simulink model "Part_b"  (R2021b)
settings: Solver=FixedStepDiscrete  StartTime=0.0  StopTime=inf  RelTol=1e-3
undefined symbols (not defined in the file): D4
libraries: androiduilib x8, androidsensorlib x2, androidaudiovideolib x1, androidcommunicationlib x1, fuzblock x1
settings Model: Creator=Nishikant Parmar  LastModifiedBy=Nishikant Parmar
settings OptimizationCC: EnhancedBackFolding=on  PassReuseOutputArgsAs=Individual arguments  ZeroExternalMemoryAtStartup=off  ZeroInternalMemoryAtStartup=off  MaxStackSize=64  OptimizeBlockOrder=speed  DifferentSizesBufferReuse=on  OptimizationCustomize=off  EfficientTunableParamExpr=on
settings DebuggingCC: ParameterTunabilityLossMsg=error
settings HardwareCC: ProdBitPerPointer=32  ProdBitPerSizeT=32  ProdBitPerPtrDiffT=32  ProdLargestAtomicInteger=Long  ProdLargestAtomicFloat=Double  ProdWordSize=32  ProdHWDeviceType=ARM Compatible->ARM Cortex  UseEmbeddedCoderFeatures=off  UseSimulinkCoderFeatures=off
settings SFSimCC: MATLABDynamicMemAlloc=off
settings RTWCC: Description=Embedded Coder  SystemTargetFile=ert.tlc  HardwareBoard=Android Device  TLCOptions="-aInlineSetEventsForThisBaseRateFcn=TLC_FALSE -aSuppressMultiTaskScheduler=TLC_FALSE  -aRateBasedStepFcn=0"  TemplateMakefile=ert_default_tmf  RTWVerbose=off  Toolchain=Android SDK/NDK Tools
settings CodeAppCC: ForceParamTrailComments=on  IgnoreCustomStorageClasses=off  OperatorAnnotations=on  SimulinkDataObjDesc=on  SFDataObjDesc=on  InsertBlockDesc=on
settings ERTTargetCC: SupportNonInlinedSFcns=on

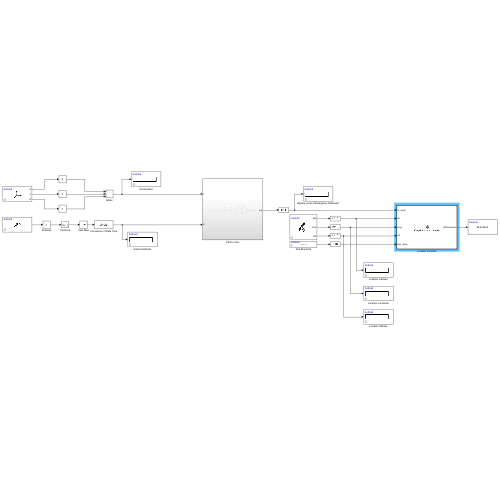
[thumbnail: Simulink's stored preview of the top-level diagram]
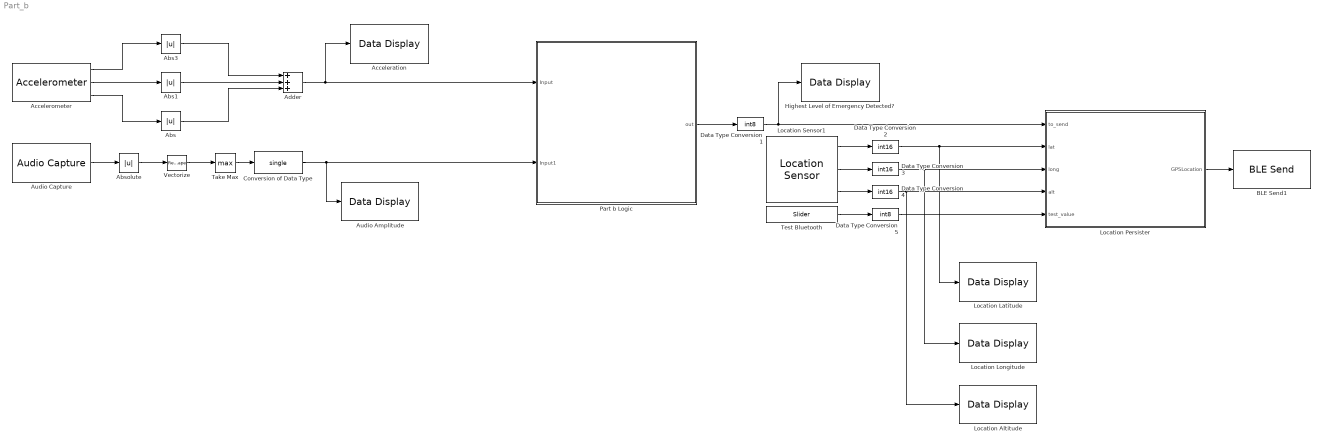
== system Part_b ==
  Abs : Abs
  Abs1 : Abs
  Abs3 : Abs
  Absolute : Abs
  Acceleration : androiduilib/Data Display  DataDisplayId=Part_b/Acceleration  Format=Float  Precision=6  SimulateUsing=Code generation  blockPlatform=Android
      settings: SourceProductBaseCode=ANDROID
  Accelerometer : androidsensorlib/Accelerometer  OutputVector=off  SampleTime=0.1  BlockPlatform=Android
      settings: SourceProductBaseCode=ANDROID
  Adder : Sum  Inputs=+++
  Audio Amplitude : androiduilib/Data Display  DataDisplayId=Part_b/Audio_Amplitude  Format=Float  Precision=6  SimulateUsing=Code generation  blockPlatform=Android
      settings: SourceProductBaseCode=ANDROID
  Audio Capture : androidaudiovideolib/Audio Capture  SampleFreq=44100  FrameSize=4410  SampleTime=0.1  SimulateUsing=Code generation  DeviceStr=0  QueueDuration=0  BlockPlatform=Android  AudioSamplingFreq=44100
      settings: SourceProductBaseCode=ANDROID
  BLE Send1 : androidcommunicationlib/BLE Send  DeviceMode=Peripheral (Server)  BluetoothAddress=D4:8A:39:6B:66:89  CharUUID=00002a05-0000-1000-8000-00805f9b34fb  ServiceUUID=00001801-0000-1000-8000-00805f9b34fb  device=Nishikant's Galaxy M31s  character=Generic Attribute\Service Changed  CustomService=off  ServiceName=Heart Rate  CharacteristicName="Heart Rate  Measurement"  CustomServiceUUID=<Enter Service UUID>  CustomCharUUID=<Enter Characteristic UUID>  charseruuid=00001801-0000-1000-8000-00805f9b34fb\00002a05-0000-1000-8000-00805f9b34fb  seruuid=00001810-0000-1000-8000-00805f9b34fb  chruuid=00002a37-0000-1000-8000-00805f9b34fb  PeripheralService=0000180d-0000-1000-8000-00805f9b34fb  PeripheralCharacteristic=00002a37-0000-1000-8000-00805f9b34fb  BLEId=Part_b/BLE_Send1  Devicename=Nishikant's Galaxy M31s  IsCustomService=0  Size=-1
      settings: SourceProductBaseCode=ANDROID
  Conversion of Data Type : DataTypeConversion  OutDataTypeStr=single
  Data Type Conversion1 : DataTypeConversion  OutDataTypeStr=int8
  Data Type Conversion2 : DataTypeConversion  OutDataTypeStr=int16
  Data Type Conversion3 : DataTypeConversion  OutDataTypeStr=int16
  Data Type Conversion4 : DataTypeConversion  OutDataTypeStr=int16
  Data Type Conversion5 : DataTypeConversion  OutDataTypeStr=int8
  Highest Level of Emergency Detected? : androiduilib/Data Display  DataDisplayId=Part_b/Highest_Level_of_Emergency_Detected?  Format=Float  Precision=6  SimulateUsing=Code generation  blockPlatform=Android
      settings: SourceProductBaseCode=ANDROID
  Location Altitude : androiduilib/Data Display  DataDisplayId=Part_b/Location_Altitude  Format=Float  Precision=6  SimulateUsing=Code generation  blockPlatform=Android
      settings: SourceProductBaseCode=ANDROID
  Location Latitude : androiduilib/Data Display  DataDisplayId=Part_b/Location_Latitude  Format=Float  Precision=6  SimulateUsing=Code generation  blockPlatform=Android
      settings: SourceProductBaseCode=ANDROID
  Location Longitude : androiduilib/Data Display  DataDisplayId=Part_b/Location_Longitude  Format=Float  Precision=6  SimulateUsing=Code generation  blockPlatform=Android
      settings: SourceProductBaseCode=ANDROID
  Location Persister : MATLAB Function  TreatAsAtomicUnit=on
  Location Sensor1 : androidsensorlib/Location Sensor  OutputVector=off  SampleTime=0.1  BlockPlatform=Android
      settings: SourceProductBaseCode=ANDROID
  Part b Logic : Subsystem
  Take Max : MinMax  Function=max
  Test Bluetooth : androiduilib/Slider  Min=-127  Value=0  Max=128  Resolution=1  SliderId=Part_b/Test_Bluetooth  SampleTime=0.1  BlockPlatform=Android
      settings: SourceProductBaseCode=ANDROID
  Vectorize : Reshape
  wires:
  Audio Capture/1 -> Absolute/1
  Accelerometer/1 -> Abs3/1
  Accelerometer/2 -> Abs1/1
  Accelerometer/3 -> Abs/1
  Abs3/1 -> Adder/1
  Abs1/1 -> Adder/2
  Abs/1 -> Adder/3
  Absolute/1 -> Vectorize/1
  Vectorize/1 -> Take Max/1
  Adder/1 -> Acceleration/1, Part b Logic/1(Input)
  Take Max/1 -> Conversion of Data Type/1
  Conversion of Data Type/1 -> Part b Logic/2(Input1), Audio Amplitude/1
  Data Type Conversion4/1 -> Location Altitude/1, Location Persister/4(alt)
  Location Sensor1/2 -> Data Type Conversion3/1
  Data Type Conversion3/1 -> Location Longitude/1, Location Persister/3(long)
  Test Bluetooth/1 -> Data Type Conversion5/1
  Location Persister/1(GPSLocation) -> BLE Send1/1
  Data Type Conversion1/1 -> Highest Level of Emergency Detected?/1, Location Persister/1(to_send)
  Data Type Conversion5/1 -> Location Persister/5(test_value)
  Data Type Conversion2/1 -> Location Latitude/1, Location Persister/2(lat)
  Part b Logic/1(out) -> Data Type Conversion1/1
  Location Sensor1/3 -> Data Type Conversion4/1
  Location Sensor1/1 -> Data Type Conversion2/1

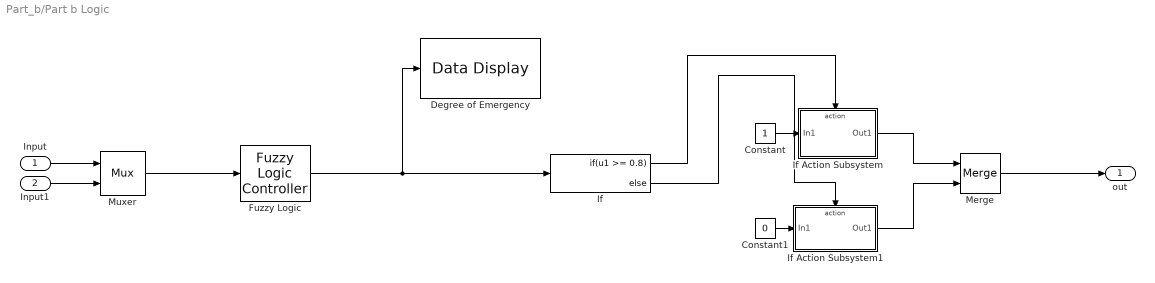
== system Part_b/Part b Logic ==
  Input : Inport
  Input1 : Inport  Port=2
  Constant : Constant
  Constant1 : Constant  Value=0
  Degree of Emergency : androiduilib/Data Display  DataDisplayId=Part_b/Part_b_Logic/Degree_of_Emergency  Format=Float  Precision=6  SimulateUsing=Code generation  blockPlatform=Android
      settings: SourceProductBaseCode=ANDROID
  Fuzzy Logic : fuzblock/Fuzzy Logic  Controller  FIS='D:\Work\Academics\Semester - 7\Nature Inspired Computing\Assignment6\FuzzyLogic.fis'  OutputSampleNumber=101  DataType=double  FuzzifiedInputs=off  RuleFiringStrengths=off  RuleOutputs=off  AggregatedOutputs=off  SimulateUsing=Interpreted execution  OutOfRangeInputValueMessage=warning  NoRuleFiredMessage=warning  EmptyOutputFuzzySetMessage=warning
  If : If  IfExpression=u1 >= 0.8
  If Action Subsystem : Subsystem  TreatAsAtomicUnit=on
  If Action Subsystem1 : Subsystem  TreatAsAtomicUnit=on
  Merge : Merge
  Muxer : Mux  Inputs=2
  out : Outport
  wires:
  If/1 -> If Action Subsystem/Action
  If Action Subsystem/1(Out1) -> Merge/1
  If/2 -> If Action Subsystem1/Action
  Constant/1 -> If Action Subsystem/1(In1)
  If Action Subsystem1/1(Out1) -> Merge/2
  Fuzzy Logic/1 -> If/1, Degree of Emergency/1
  Constant1/1 -> If Action Subsystem1/1(In1)
  Merge/1 -> out/1
  Input/1 -> Muxer/1
  Input1/1 -> Muxer/2
  Muxer/1 -> Fuzzy Logic/1

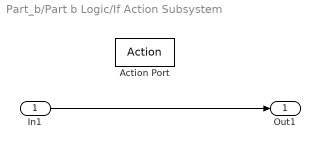
== system Part_b/Part b Logic/If Action Subsystem ==
  In1 : Inport
  Action Port : ActionPort  ActionPortLabel=if(u1 >= 0.8)
  Out1 : Outport
  wires:
  In1/1 -> Out1/1

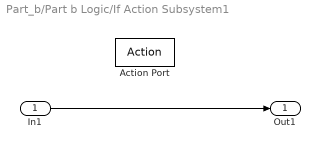
== system Part_b/Part b Logic/If Action Subsystem1 ==
  In1 : Inport
  Action Port : ActionPort  ActionPortLabel=else
  Out1 : Outport
  wires:
  In1/1 -> Out1/1

== matlab function Part_b/Location Persister ==
  data: to_send input; lat input; GPSLocation output; long input; alt input; test_value input
function GPSLocation = KeepPersistentLocation(to_send, lat, long, alt, test_value)

% Reference - https://in.mathworks.com/matlabcentral/answers/11323-hold-true-value-for-finite-length-of-time

persistent  lat_value long_value alt_value;

if isempty(lat_value)          
     lat_value = int16(0);
end

if isempty(long_value)     
     long_value = int16(0);
end

if isempty(alt_value)
     alt_value = int16(0);
end

if to_send == 1    
    lat_value = lat;
    long_value = long;
    alt_value = alt;
end


GPSLocation = zeros(7,1,'uint8');
[lower_lat, upper_lat] = getBytesInTwoHalves(lat_value);
[lower_long, upper_long] = getBytesInTwoHalves(long_value);
[lower_alt, upper_alt] = getBytesInTwoHalves(alt_value);
GPSLocation(1) = uint8(bin2dec(dec2bin(test_value, 8)));
GPSLocation(2) = lower_lat;
GPSLocation(3) = upper_lat;
GPSLocation(4) = lower_long;
GPSLocation(5) = upper_long;
GPSLocation(6) = lower_alt;
GPSLocation(7) = upper_alt;

end

function [lower,upper] = getBytesInTwoHalves(decimal)
binary = dec2bin(int16(decimal),16);
lower = uint8(bin2dec(binary(9:16)));
upper= uint8(bin2dec(binary(1:8)));
end
